simulink model "NCO"  (R2023b)
settings: Solver=FixedStepAuto  StartTime=0.0  StopTime=1  MaxStep=1e-8  RelTol=1e-3
libraries: hdlsllib x1, dsphdlsigops2 x1
settings Model: Creator=31651  LastModifiedBy=31651
settings OptimizationCC: BlockReduction=off  ConditionallyExecuteInputs=off  DefaultParameterBehavior=Inlined
settings DebuggingCC: AlgebraicLoopMsg=error  ParameterOverflowMsg=none
settings HardwareCC: ProdBitPerPointer=32  ProdBitPerSizeT=32  ProdBitPerPtrDiffT=32  ProdLargestAtomicFloat=None  ProdIntDivRoundTo=Undefined  ProdEndianess=Unspecified  ProdWordSize=32  ProdHWDeviceType=ASIC/FPGA->ASIC/FPGA  TargetBitPerPointer=64  TargetBitPerSizeT=64  TargetBitPerPtrDiffT=64  TargetLongLongMode=on  TargetIntDivRoundTo=Zero  TargetEndianess=LittleEndian  TargetWordSize=64  TargetHWDeviceType=Custom Processor->MATLAB Host Computer  ProdEqTarget=off

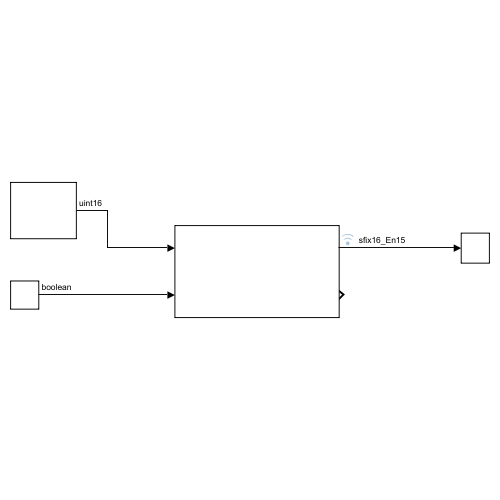
[thumbnail: Simulink's stored preview of the top-level diagram]
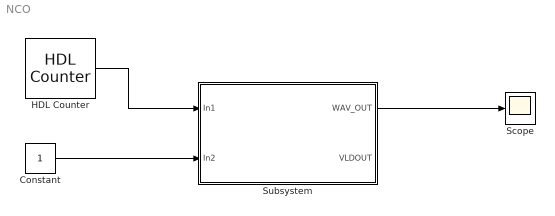
== system NCO ==
  Constant : Constant  OutDataTypeStr=boolean
  HDL Counter : hdlsllib/Sources/HDL Counter  CountType=Free running  CountInit=1  CountStep=655  CountMax=25  CountFromType=Initial value  CountFrom=1  CountResetPort=off  CountLoadPort=off  CountEnbPort=off  CountDirPort=off  CountHitOutputPort=off  CountDataType=Unsigned  CountWordLen=16  CountFracLen=0  CountSampTime=1
  Scope : Scope
  Subsystem : Subsystem
  wires:
  HDL Counter/1 -> Subsystem/1(In1)
  Constant/1 -> Subsystem/2(In2)
  Subsystem/1(WAV_OUT) -> Scope/1

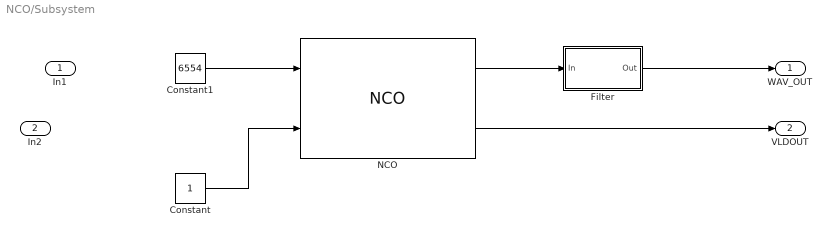
== system NCO/Subsystem ==
  In1 : Inport
  In2 : Inport  Port=2
  Constant : Constant  OutDataTypeStr=boolean  SampleTime=1/100000
  Constant1 : Constant  Value=6554  SampleTime=1/100000
  Filter : Subsystem  Tag=BlockMethodSubSystem
  NCO : dsphdlsigops2/NCO  PhaseIncrementSource=Input port  PhaseIncrement=100  PhaseOffsetSource=Property  PhaseOffset=0  DitherSource=Property  NumDitherBits=4  SamplesPerFrame=1  LUTCompress=off  ResetAction=off  Waveform=Sine  PhasePort=off  SimulateUsing=Code generation  AccumulatorWL=16  PhaseQuantization=on  NumQuantizerAccumulatorBits=12  OutputDataType=Binary point scaling  OutputWL=16  OutputFL=15
      settings: LibrarySourceBlock=dsphdlsrcs2/NCO
  WAV_OUT : Outport
  VLDOUT : Outport  Port=2
  wires:
  NCO/2 -> VLDOUT/1
  NCO/1 -> Filter/1(In)
  Filter/1(Out) -> WAV_OUT/1
  Constant/1 -> NCO/2
  Constant1/1 -> NCO/1

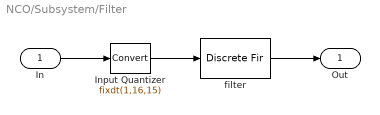
== system NCO/Subsystem/Filter ==
  In : Inport
  Input Quantizer : DataTypeConversion  OutDataTypeStr=fixdt(1,16,15)  RndMeth=Round
  filter : DiscreteFir  Coefficients=[-0.000613535726833574352 0.00039610627927773171 -7.85646380987156457e-18 -0.000477198755296996788 0.000879639178195992886 -0.00101764246035848118 0.000734305574276288941 5.74433321343095593e-18 -0.00101049560227826018 0.00191593147758841505 -0.00223842673678539958 0.00161009807669441028 -3.11094400855593708e-17 -0.00215299220919710653 0.00400215318464021679 -0.00457889929662995149 0.00322524673062784661 -1.37366680307676234e-17 -0.00414661320195481437 0.00757447010187824697 -0.00853100164817993493 0.00592694297089688734 -1.94065078789124378e-17 -0.00746150421198605793 0.0135351534289510651 -0.0151788712791869913 0.0105310756055852477 -2.46775718744965288e-17 -0.0133601486975479678 0.0244858153050784948 -0.0278961439264566041 0.0197977666609277791 -2.87272140703832377e-17 -0.0270720885837576267 0.0526931254016028 -0.0653562638534140317 0.0525450732153632249 -3.09234137317473368e-17 -0.124407267360874429 0.60564619035915368 0.60564619035915368 -0.124407267360874429 -3.09234137317473368e-17 0.0525450732153632249 -0.0653562638534140317 0.0526931254016028 -0.0270720885837576267 -2.87272140703832377e-17 0.0197977666609277791 -0.0278961439264566041 0.0244858153050784948 -0.0133601486975479678 -2.46775718744965288e-17 0.0105310756055852477 -0.0151788712791869913 0.0135351534289510651 -0.00746150421198605793 -1.94065078789124378e-17 0.00592694297089688734 -0.00853100164817993493 0.00757447010187824697 -0.00414661320195481437 -1.37366680307676234e-17 0.00322524673062784661 -0.00457889929662995149 0.00400215318464021679 -0.00215299220919710653 -3.11094400855593708e-17 0.00161009807669441028 -0.00223842673678539958 0.00191593147758841505 -0.00101049560227826018 5.74433321343095593e-18 0.000734305574276288941 -0.00101764246035848118 0.000879639178195992886 -0.000477198755296996788 -7.85646380987156457e-18 0.00039610627927773171 -0.000613535726833574352]  InputProcessing=Columns as channels (frame based)  CoefDataTypeStr=fixdt(false,16,16)  ProductDataTypeStr=fixdt(true,31,30)  AccumDataTypeStr=fixdt(true,33,30)  OutDataTypeStr=fixdt(true,16,15)  RndMeth=Convergent
  Out : Outport
  wires:
  In/1 -> Input Quantizer/1
  Input Quantizer/1 -> filter/1
  filter/1 -> Out/1
